simulink model "LQRSimulink"  (R2025b)
settings: Solver=VariableStepAuto  StartTime=0.0  StopTime=100  RelTol=1e-3
values from neighbouring files (symbols this model uses):
  B_ctrl = B_long(:, 1:3)    [LQRAnalysis.m]    (also in LQRclassic.m)
undefined symbols (not defined in the file or in its folder): A_long, K
settings Model: Creator=leonardoleggeri  LastModifiedBy=leonardoleggeri

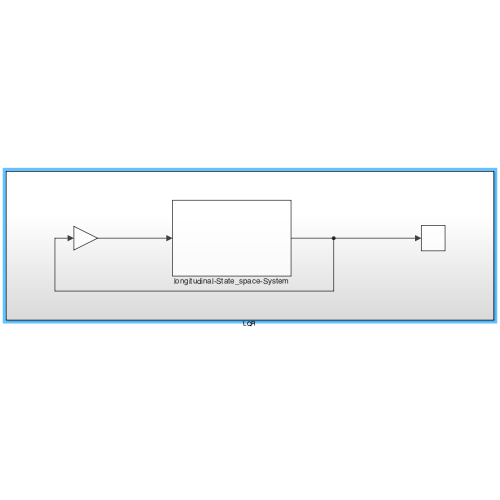
[thumbnail: Simulink's stored preview of the top-level diagram]
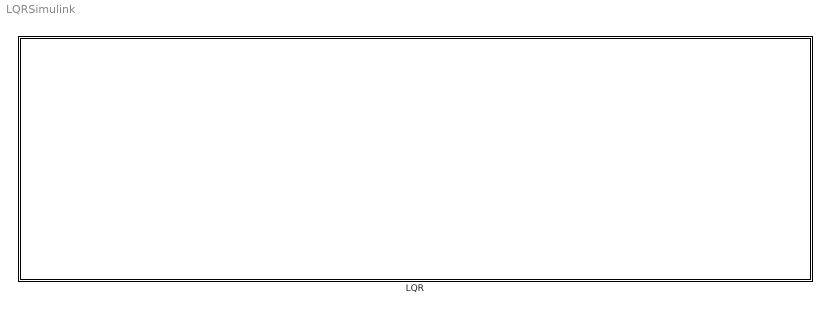
== system LQRSimulink ==
  LQR : Subsystem

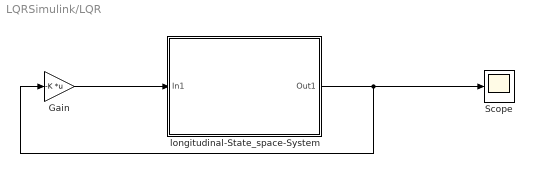
== system LQRSimulink/LQR ==
  Gain : Gain  Gain=-K  Multiplication=Matrix(K*u)
  Scope : Scope
      settings: ActiveDisplayYMinimum=-15.105471283201926  ActiveDisplayYMaximum=7.7125068715165925
  longitudinal-State_space-System : Subsystem
      mask Display: image('F16_SCANG_InFlight.jpg');
  wires:
  Gain/1 -> longitudinal-State_space-System/1(In1)
  longitudinal-State_space-System/1(Out1) -> Scope/1, Gain/1

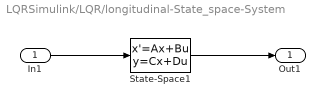
== system LQRSimulink/LQR/longitudinal-State_space-System ==
  In1 : Inport
  State-Space1 : StateSpace  A=A_long  B=B_ctrl  C=eye(4)  D=zeros(4,3)  InitialCondition=[0.8; 0.6; 50; 15]
  Out1 : Outport
  wires:
  In1/1 -> State-Space1/1
  State-Space1/1 -> Out1/1
